simulink model "DIC_control"  (R2021a)
settings: Solver=VariableStepAuto  StartTime=0.0  StopTime=T  RelTol=1e-3
values from neighbouring files (symbols this model uses):
  a = ksi * ksi * 0.25 * 2    (= 2)    [phase_portrait2.m]    (also in phase_portrait_ex2.m = 8; plot_ex1.m = 8; smc_ex2.m)
  b = v2(2) - m * v2(1)    [phase_portrait2.m]    (also in phase_portrait_ex2.m = 0; plot_ex1.m = 15)
  c = 10    [phase_portrait_ex2.m]    (also in plot_ex1.m; smc_ex2.m = -0.732050807569)
  dist = 1    [plot_ex1.m]
  h = 300    [plot_ex1.m]
  K = 4    [plot_ex1.m]
  lambda = 20    [plot_ex1.m]
  ss_st = 0.0001    [plot_ex1.m]
  yd = 2    [plot_ex1.m]
  ydd = 0    [plot_ex1.m]
settings Model: Creator=root  LastModifiedBy=root
settings SolverCC: ZeroCrossAlgorithm=Adaptive
settings DebuggingCC: MaxConsecutiveZCsMsg=none  IgnoredZcDiagnostic=none

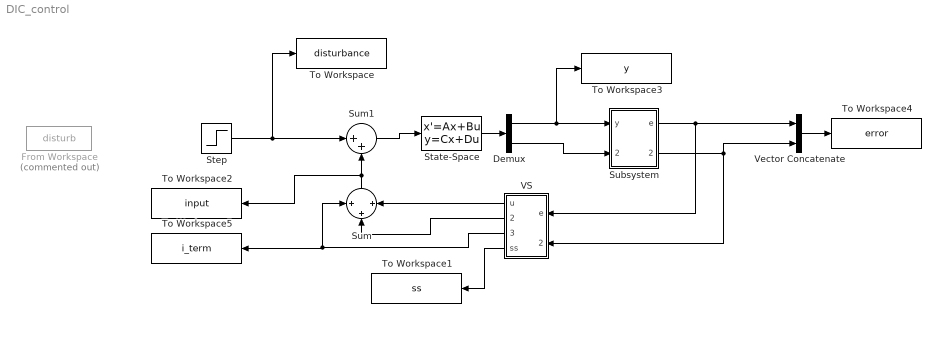
== system DIC_control ==
  Demux : Demux  Outputs=2
  From Workspace : FromWorkspace  Commented=on  VariableName=disturb  SampleTime=0.0001
  State-Space : StateSpace  A=[0 1; -b -a]  B=[0; 1]  C=eye(2)  D=zeros(2, 1)  InitialCondition=[0 0]
  Step : Step  After=dist  SampleTime=ss_st  ZeroCross=off
  Subsystem : Subsystem
  Sum : Sum  Inputs=+|+|+
  Sum1 : Sum  Inputs=|++
  To Workspace : ToWorkspace  VariableName=disturbance  SaveFormat=Timeseries  SampleTime=-1
  To Workspace1 : ToWorkspace  VariableName=ss  SaveFormat=Timeseries  SampleTime=-1
  To Workspace2 : ToWorkspace  VariableName=input  SaveFormat=Timeseries  SampleTime=-1
  To Workspace3 : ToWorkspace  VariableName=y  SaveFormat=Timeseries  SampleTime=-1
  To Workspace4 : ToWorkspace  VariableName=error  SaveFormat=Timeseries  SampleTime=-1
  To Workspace5 : ToWorkspace  VariableName=i_term  SaveFormat=Timeseries  SampleTime=-1
  VS : Subsystem
  Vector Concatenate : Concatenate
  wires:
  Demux/2 -> Subsystem/2(ydot)
  Vector Concatenate/1 -> To Workspace4/1
  State-Space/1 -> Demux/1
  Subsystem/2(edot) -> VS/2(edot), Vector Concatenate/2
  Demux/1 -> To Workspace3/1, Subsystem/1(y)
  VS/4(ss) -> To Workspace1/1
  Subsystem/1(e) -> VS/1(e), Vector Concatenate/1
  Sum1/1 -> State-Space/1
  Sum/1 -> To Workspace2/1, Sum1/2
  VS/1(u) -> Sum/3
  VS/2(p_term) -> Sum/2
  VS/3(i_term) -> To Workspace5/1, Sum/1
  Step/1 -> To Workspace/1, Sum1/1

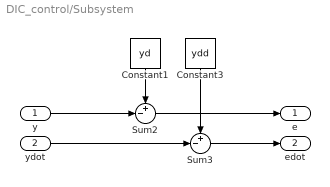
== system DIC_control/Subsystem ==
  y : Inport
  ydot : Inport  Port=2
  Constant1 : Constant  Value=yd
  Constant3 : Constant  Value=ydd
  Sum2 : Sum  Inputs=+-|
  Sum3 : Sum  Inputs=+-|
  e : Outport
  edot : Outport  Port=2
  wires:
  Constant1/1 -> Sum2/1
  Sum2/1 -> e/1
  Constant3/1 -> Sum3/1
  Sum3/1 -> edot/1
  ydot/1 -> Sum3/2
  y/1 -> Sum2/2

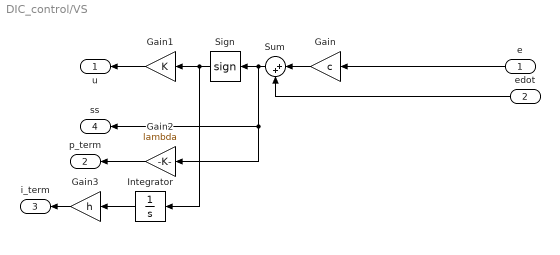
== system DIC_control/VS ==
  e : Inport
  edot : Inport  Port=2
  Gain : Gain  Gain=c
  Gain1 : Gain  Gain=K
  Gain2 : Gain  Gain=lambda
  Gain3 : Gain  Gain=h
  Integrator : Integrator
  Sign : Signum
  Sum : Sum  Inputs=|++
  u : Outport
  p_term : Outport  Port=2
  i_term : Outport  Port=3
  ss : Outport  Port=4
  wires:
  Sign/1 -> Integrator/1, Gain1/1
  Gain/1 -> Sum/1
  e/1 -> Gain/1
  Sum/1 -> Gain2/1, ss/1, Sign/1
  edot/1 -> Sum/2
  Gain1/1 -> u/1
  Gain2/1 -> p_term/1
  Integrator/1 -> Gain3/1
  Gain3/1 -> i_term/1
